simulink model "COMPoseTesting"  (Simulink 7.9)
settings: Solver=ode3  StartTime=0.0  StopTime=inf  FixedStep=1  RelTol=1e-3
libraries: simulink x1
settings Model: Creator=jorhabib  LastModifiedBy=jorhabib

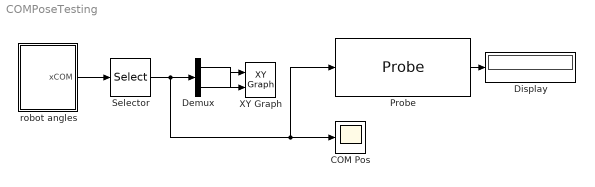
== system COMPoseTesting ==
  COM Pos : Scope
      settings: TimeRange=500  YMin=-0.07  YMax=0.07
  Demux : Demux  Outputs=2
  Display : Display
  Probe : Probe  ProbeWidth=off  ProbeComplexSignal=off
  Selector : Selector  InputPortWidth=7  IndexOptions=Index vector (dialog)  Indices=[1:2]  OutputSizes=1
  XY Graph : simulink/Sinks/XY Graph  xmin=-0.1  xmax=0.01  ymin=-0.05  ymax=0.05  st=-1
  robot angles : Subsystem
  wires:
  robot angles/1(xCOM) -> Selector/1
  Selector/1 -> Demux/1, COM Pos/1, Probe/1
  Demux/2 -> XY Graph/1
  Demux/1 -> XY Graph/2
  Probe/1 -> Display/1

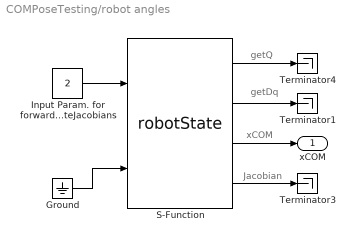
== system COMPoseTesting/robot angles ==
  note: Jacobian
  note: getQ
  note: xCOM
  note: getDq
  Ground : Ground
  "Input Param. for forwardKinematics and  computeJacobians " : Constant  Value=2  OutDataTypeStr=int8
  S-Function : S-Function  FunctionName=robotState  Parameters=val,robotname,localname  EnableBusSupport=off  mask{val=2, robotname='icubSim', localname='robotState'}
      mask prompts: val "Value"; robotname "Robot Name (icub - icubSim)"; localname "Module Name"
  Terminator1 : Terminator
  Terminator3 : Terminator
  Terminator4 : Terminator
  xCOM : Outport
  wires:
  S-Function/4 -> Terminator3/1
  "Input Param. for forwardKinematics and  computeJacobians "/1 -> S-Function/1
  S-Function/3 -> xCOM/1
  S-Function/1 -> Terminator4/1
  S-Function/2 -> Terminator1/1
  Ground/1 -> S-Function/2
